simulink model "Block_FI"  (R2022a)
settings: Solver=ode23tb  StartTime=0.0  StopTime=0.03  MaxStep=1e-4  RelTol=1e-5
undefined symbols (not defined in the file): FI
libraries: simulink x1
settings Model: Creator=админ  LastModifiedBy=админ

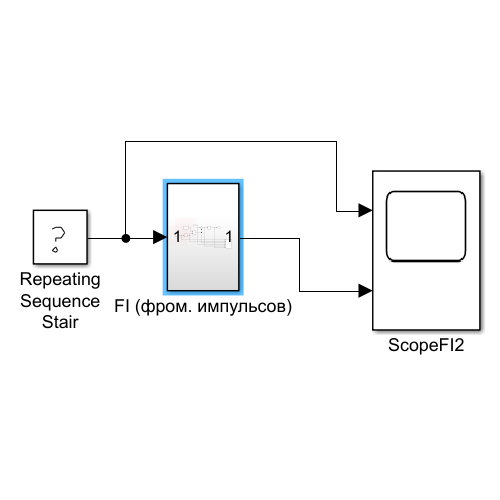
[thumbnail: Simulink's stored preview of the top-level diagram]
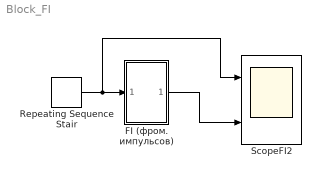
== system Block_FI ==
  FI (фром. импульсов) : Subsystem
  Repeating Sequence Stair : simulink/Sources/Repeating Sequence Stair  OutValues=FI.RSS_Vector  tsamp=FI.RSS_st  OutMin=[]  OutMax=[]  OutDataTypeStr=double  OutputDataTypeScalingMode=double  OutDataType=fixdt(0,8)  ConRadixGroup=Best Precision: Vector-wise  OutScaling=2^-12
  ScopeFI2 : Scope  NumInputPorts=2
  wires:
  Repeating Sequence Stair/1 -> ScopeFI2/1, FI (фром. импульсов)/1(In1)
  FI (фром. импульсов)/1(Out1) -> ScopeFI2/2

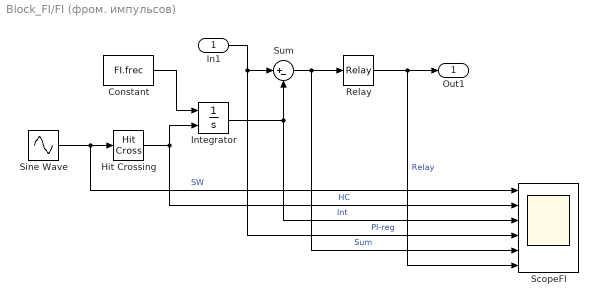
== system Block_FI/FI (фром. импульсов) ==
  In1 : Inport
  Constant : Constant  Value=FI.frec
  Hit Crossing : HitCross
  Integrator : Integrator  ExternalReset=rising
  Relay : Relay
  ScopeFI : Scope  NumInputPorts=6
  Sine Wave : Sin  Frequency=FI.Sine_Wave.freq  SampleTime=0
  Sum : Sum  Inputs=|+-
  Out1 : Outport
  wires:
  Sine Wave/1 -> ScopeFI/1, Hit Crossing/1  "SW"
  Relay/1 -> Out1/1, ScopeFI/6  "Relay"
  In1/1 -> ScopeFI/4, Sum/1  "PI-reg"
  Hit Crossing/1 -> ScopeFI/2, Integrator/2  "HC"
  Integrator/1 -> ScopeFI/3, Sum/2  "Int"
  Constant/1 -> Integrator/1
  Sum/1 -> ScopeFI/5, Relay/1  "Sum"
